simulink model "pv_mpp"  (R2023b)
settings: Solver=VariableStepAuto  StartTime=0.0  StopTime=10.0  RelTol=1e-3
libraries: spsSeriesRLCBranchLib x4, spsCurrentMeasurementLib x1, spsDiodeLib x1, spsIGBTDiodeLib x1, spsPVArrayLib x1, spsPWMGeneratorDCDCLib x1, spsVoltageMeasurementLib x1, sps_lib x1
settings Model: Creator=SAUMYA  LastModifiedBy=SAUMYA

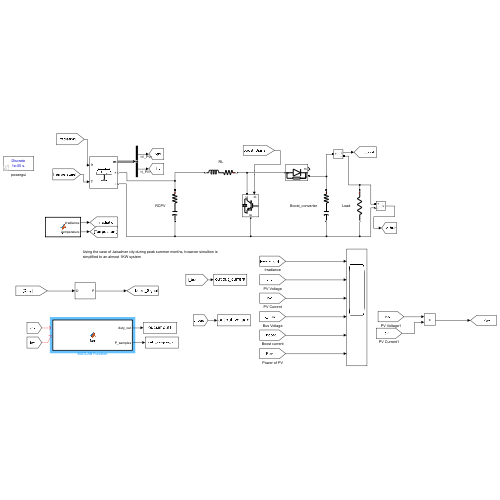
[thumbnail: Simulink's stored preview of the top-level diagram]
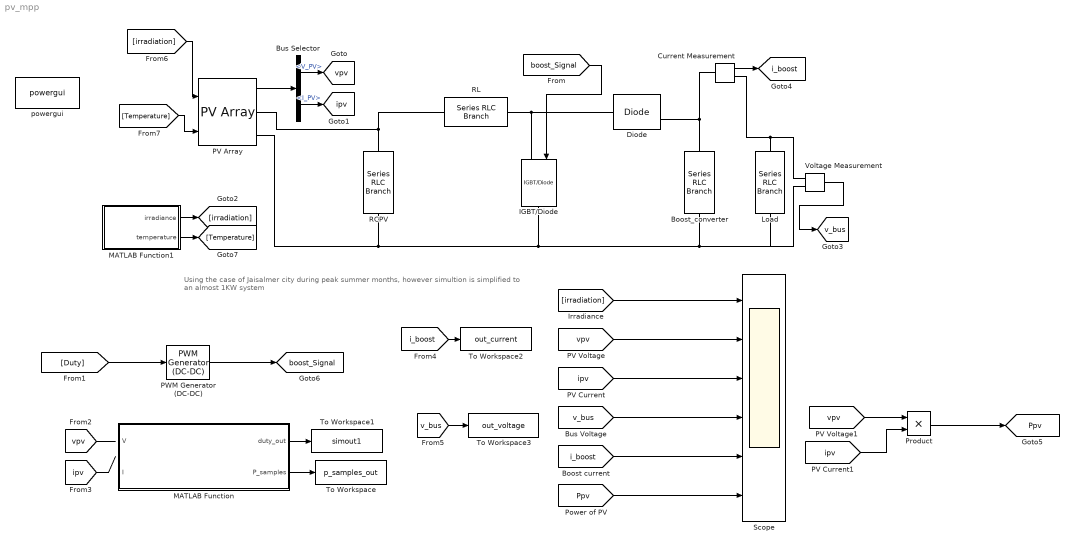
== system pv_mpp ==
  note: Using the case of Jaisalmer city during peak summer months, however simultion is simplified to an almost 1KW system
  Boost_converter : spsSeriesRLCBranchLib/Series RLC Branch  LConnTagsString=__new0  RConnTagsString=__new0  BranchType=RC  Resistance=1e-4  Inductance=1e-3  SetiL0=off  InitialCurrent=0  Capacitance=3300e-6  Setx0=on  InitialVoltage=0  Measurements=None
  Bus Selector : BusSelector  OutputSignals=V_PV,I_PV
  Current Measurement : spsCurrentMeasurementLib/Current Measurement  PhasorSimulation=off  OutputType=Complex  PSBequivalent=0
  Diode : spsDiodeLib/Diode  Ron=0.001  Lon=0  Vf=0.8  IC=0  UseSnubber=0  Rs=500  Cs=250e-9  Measurements=on
  IGBT/Diode : spsIGBTDiodeLib/IGBT//Diode  Ron=1e-3  Rs=1e5  Cs=inf  Measurements=off
  Load : spsSeriesRLCBranchLib/Series RLC Branch  LConnTagsString=__new0  RConnTagsString=__new0  BranchType=R  Resistance=10  Inductance=1e-3  SetiL0=off  InitialCurrent=0  Capacitance=3300e-6  Setx0=on  InitialVoltage=0  Measurements=None
  MATLAB Function : MATLAB Function  TreatAsAtomicUnit=on
  MATLAB Function1 : MATLAB Function  TreatAsAtomicUnit=on
  PV Array : spsPVArrayLib/PV Array  Npar=5  Nser=1  PlotType=array @ 1000 W/m2 & specified temperatures  S_vec="[ 1000  500  100 ]"  Temp_C_vec=[ 15 25 35 45 55 ]  ModuleName=Changzhou Almaden SEBP60S-220  PlotWhenSelected=off  Pm=219.876  Ncell=60  Voc=36.06  Isc=7.95  Vm=30.12  Im=7.3  beta_Voc_pc=-0.3624  alpha_Isc_pc=0.054805  beta_Voc=-0.13068  alpha_Isc=0.004357  IL=7.9642  I0=2.8692e-10  nI=0.97455  Rsh=106.1817  Rs=0.18964  RobustModel=off  RobustCellTemperature=313.3991  BAL=on  Tc=1e-6  Tfilter=5e-5
  PWM Generator (DC-DC) : spsPWMGeneratorDCDCLib/PWM Generator (DC-DC)  Fsw=5000  Ts=10e-3
  Product : Product
  RCPV : spsSeriesRLCBranchLib/Series RLC Branch  LConnTagsString=__new0  RConnTagsString=__new0  BranchType=RC  Resistance=1e-4  Inductance=1e-3  SetiL0=off  InitialCurrent=0  Capacitance=100e-6  Setx0=on  InitialVoltage=0  Measurements=None
  RL : spsSeriesRLCBranchLib/Series RLC Branch  LConnTagsString=__new0  RConnTagsString=__new0  BranchType=RL  Resistance=0.1  Inductance=1e-3  SetiL0=off  InitialCurrent=0  Capacitance=1e-3  Setx0=on  InitialVoltage=0  Measurements=None
  Scope : Scope  NumInputPorts=6
  To Workspace : ToWorkspace  VariableName=p_samples_out  SaveFormat=Structure With Time  SampleTime=-1
  To Workspace1 : ToWorkspace  VariableName=simout1  SaveFormat=Structure With Time  SampleTime=-1
  To Workspace2 : ToWorkspace  VariableName=out_current  SaveFormat=Structure With Time  SampleTime=-1
  To Workspace3 : ToWorkspace  VariableName=out_voltage  SaveFormat=Structure With Time  SampleTime=-1
  Voltage Measurement : spsVoltageMeasurementLib/Voltage Measurement  PhasorSimulation=off  OutputType=Complex  PSBequivalent=0
  powergui : sps_lib/powergui  Priority=1  SimulationMode=Discrete  SampleTime=1e-05  frequency=60  Iterations=50  frequencyindice=0  Pbase=100e6  ErrMax=1e-4  UnitsV=kV  UnitsW=MW  buscounter=0  FunctionMessages=off  echomessages=off  EnableUseOfTLC=off  CurrentSourceSwitches=off  DisableSnubberDevices=off  DisableRonSwitches=off  DisableVfSwitches=off  DisplayEquations=off  AutomaticDiscreteSolvers=off  SolverType=Tustin/Backward Euler (TBE)  Interpol=off  ExternalGateDelay=off  methode=off  Ts=100  x0status=blocks  SPID=on  SwTol=0  HookPort=off  NonlinearTolerance=1e-4  nMaxIteration=100  ContinueOnMaxIteration=off  RestoreLinks=warning  ResistiveCurrentMeasurement=off  Frange=[0:2:500]  Ylog=off  Xlog=on  ShowGrid=off  save=off  variable=ZData  structure=0  ZoomFFT=off  StartTime=0.0  cycles=1  DisplayStyle=1  fundamental=60  FreqAxis=off  MaxFrequency=1000  frequencyindicesteady=1  RmsSteady=1  display=off
  tag scope: Ppv=global, boost_Signal=global, i_boost=global, ipv=global, v_bus=global, vpv=global
  wires:
  PV Array/1 -> Bus Selector/1
  Bus Selector/2 -> [ipv]  "<I_PV>"
  Bus Selector/1 -> [vpv]  "<V_PV>"
  [boost_Signal] -> IGBT/Diode/1
  Voltage Measurement/1 -> [v_bus]
  Current Measurement/1 -> [i_boost]
  [irradiation] -> Scope/1
  [vpv] -> Scope/2
  [ipv] -> Scope/3
  [v_bus] -> Scope/4
  [i_boost] -> Scope/5
  [Ppv] -> Scope/6
  Product/1 -> [Ppv]
  [vpv] -> Product/1
  [ipv] -> Product/2
  PWM Generator (DC-DC)/1 -> [boost_Signal]
  [Duty] -> PWM Generator (DC-DC)/1
  [vpv] -> ?
  [ipv] -> ?
  MATLAB Function/2(P_samples) -> To Workspace/1
  MATLAB Function/1(duty_out) -> To Workspace1/1
  [i_boost] -> To Workspace2/1
  [v_bus] -> To Workspace3/1
  [irradiation] -> PV Array/1
  [Temperature] -> PV Array/2
  MATLAB Function1/1(irradiance) -> [irradiation]
  MATLAB Function1/2(temperature) -> [Temperature]
  connections:
  RCPV/LConn1 -- RL/RConn1 -- PV Array/RConn1
  RCPV/RConn1 -- Load/RConn1 -- Voltage Measurement/LConn2 -- Boost_converter/RConn1 -- IGBT/Diode/RConn1 -- PV Array/RConn2
  RL/LConn1 -- IGBT/Diode/LConn1 -- Diode/LConn1
  Load/LConn1 -- Voltage Measurement/LConn1 -- Current Measurement/RConn1
  Current Measurement/LConn1 -- Diode/RConn1 -- Boost_converter/LConn1

== matlab function pv_mpp/MATLAB Function1 ==
  data: irradiance output; temperature output
function [irradiance, temperature] = fcn()
%#codegen
[irradiance, temperature] = GenerateInputs();
end

== matlab function pv_mpp/MATLAB Function ==
  data: duty_out output; P_samples output; V input; I input
function [duty_out, P_samples] = fcn(V,I)
%#codegen

[duty_out, P_samples] = po_mppt(V,I);
end
